simulink model "inv_pend_delay"  (R2021b)
settings: Solver=ode45  StartTime=0.0  StopTime=8  RelTol=1e-3  EnableMultiTasking=on
settings Model: Creator=mengg_000  LastModifiedBy=1412
settings SolverCC: AlgebraicLoopSolver=TrustRegion
settings DataIOCC: LimitDataPoints=on  SaveFormat=Array  SignalLoggingSaveFormat=ModelDataLogs  ReturnWorkspaceOutputs=off
settings OptimizationCC: ExpressionDepthLimit=2147483647  LifeSpan=inf
settings DebuggingCC: UnderspecifiedInitializationDetection=Classic  MergeDetectMultiDrivingBlocksExec=none  SolverPrmCheckMsg=warning  FcnCallInpInsideContextMsg=warning  StateNameClashWarn=warning  SFUnexpectedBacktrackingDiag=warning  SFNoUnconditionalDefaultTransitionDiag=warning  SFExecutionAtInitializationDiag=none  SFMachineParentedDataDiag=warning  ArithmeticOperatorsInVariantConditions=warning
settings HardwareCC: ProdBitPerPointer=32  ProdBitPerSizeT=32  ProdBitPerPtrDiffT=32  ProdLargestAtomicFloat=None  ProdIntDivRoundTo=Undefined  ProdEndianess=Unspecified  ProdWordSize=32  ProdHWDeviceType=32-bit Generic
settings ModelReferenceCC: PropagateSignalLabelsOutOfModel=off
settings SFSimCC: SimUseLocalCustomCode=off  CustomCodeUndefinedFunction=UseInterfaceOnly
settings RTWCC: RTWUseLocalCustomCode=off
settings CodeAppCC: StateflowObjectComments=on
settings GRTTargetCC: TargetLangStandard=C89/C90 (ANSI)  CombineOutputUpdateFcns=off  GRTInterface=on
settings ConfigComp: CovMetricSettings=dw  CovSaveCumulativeToWorkspaceVar=on  CovSaveSingleToWorkspaceVar=on  CovExternalEMLEnable=off

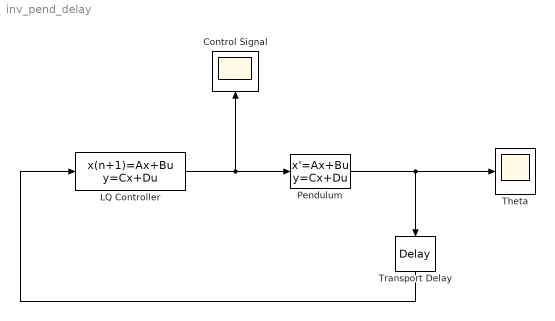
== system inv_pend_delay ==
  Control Signal : Scope
  LQ Controller : DiscreteStateSpace  A=|  B=|  C="[-12.1798  -13.3262         0]"  D=-8.1263  InitialCondition="[0;    0;   0]"  SampleTime=0.02
      A=|
      | [0.0389   -1.5001         0;
      |     0.0828    0.3594         0;
      |   -12.1798  -13.3262         0]
      B=|
      | [ -0.4344;
      |     0.1355;
      |    -8.1263]
  "Pendulum " : StateSpace  A=[0 3.0628;32 0]  B=[2; 0]  C=[0 1.5314]  D=0  InitialCondition=[0; 0.1]
  Theta : Scope
  Transport Delay : TransportDelay  DelayTime=0.04
  wires:
  "Pendulum "/1 -> Transport Delay/1, Theta/1
  Transport Delay/1 -> LQ Controller/1
  LQ Controller/1 -> "Pendulum "/1, Control Signal/1
